simulink model "PID_MODEL"  (R2023b)
settings: Solver=FixedStepDiscrete  StartTime=0.0  StopTime=50  FixedStep=0.001  RelTol=1e-3
values from neighbouring files (symbols this model uses):
  ANG_A_D_CH1_1 = 0    [ini.m]
  ANG_A_D_CH1_2 = 0    [ini.m]
  ANG_A_D_CH1_3 = 0    [ini.m]
  ANG_A_D_CH1_4 = 0    [ini.m]
  ANG_A_D_CH1_5 = 0    [ini.m]
  ANG_A_D_CH1_6 = 0    [ini.m]
  ANG_A_D_CH1_7 = 0    [ini.m]
  ANG_A_D_CH2_1 = 0    [ini.m]
  ANG_A_D_CH2_2 = 0    [ini.m]
  ANG_A_D_CH2_3 = 0    [ini.m]
  ANG_A_D_CH2_4 = 0    [ini.m]
  ANG_A_D_CH2_5 = 0    [ini.m]
  ANG_A_D_CH2_6 = 0    [ini.m]
  ANG_A_D_CH2_7 = 0    [ini.m]
  ANG_A_I_CH1_1 = 0    [ini.m]
  ANG_A_I_CH1_2 = 0    [ini.m]
  ANG_A_I_CH1_3 = 0    [ini.m]
  ANG_A_I_CH1_4 = 0    [ini.m]
  ANG_A_I_CH1_5 = 0    [ini.m]
  ANG_A_I_CH1_6 = 0    [ini.m]
  ANG_A_I_CH1_7 = 0    [ini.m]
  ANG_A_I_CH2_1 = 0    [ini.m]
  ANG_A_I_CH2_2 = 0    [ini.m]
  ANG_A_I_CH2_3 = 0    [ini.m]
  ANG_A_I_CH2_4 = 0    [ini.m]
  ANG_A_I_CH2_5 = 0    [ini.m]
  ANG_A_I_CH2_6 = 0    [ini.m]
  ANG_A_I_CH2_7 = 0    [ini.m]
  ANG_A_P_CH1_1 = 0    [ini.m]
  ANG_A_P_CH1_2 = 0    [ini.m]
  ANG_A_P_CH1_3 = 0    [ini.m]
  ANG_A_P_CH1_4 = 0    [ini.m]
  ANG_A_P_CH1_5 = 0    [ini.m]
  ANG_A_P_CH1_6 = 0    [ini.m]
  ANG_A_P_CH1_7 = 0    [ini.m]
  ANG_A_P_CH2_1 = 0    [ini.m]
  ANG_A_P_CH2_2 = 0    [ini.m]
  ANG_A_P_CH2_3 = 0    [ini.m]
  ANG_A_P_CH2_4 = 0    [ini.m]
  ANG_A_P_CH2_5 = 0    [ini.m]
  ANG_A_P_CH2_6 = 0    [ini.m]
  ANG_A_P_CH2_7 = 0    [ini.m]
  ANG_S_D_CH1_1 = 0    [ini.m]
  ANG_S_D_CH1_2 = 0    [ini.m]
  ANG_S_D_CH1_3 = 0    [ini.m]
  ANG_S_D_CH1_4 = 0    [ini.m]
  ANG_S_D_CH1_5 = 0    [ini.m]
  ANG_S_D_CH1_6 = 0    [ini.m]
  ANG_S_D_CH1_7 = 0    [ini.m]
  ANG_S_D_CH2_1 = 0    [ini.m]
  ANG_S_D_CH2_2 = 0    [ini.m]
  ANG_S_D_CH2_3 = 0    [ini.m]
  ANG_S_D_CH2_4 = 0    [ini.m]
  ANG_S_D_CH2_5 = 0    [ini.m]
  ANG_S_D_CH2_6 = 0    [ini.m]
  ANG_S_D_CH2_7 = 0    [ini.m]
  ANG_S_I_CH1_1 = 0    [ini.m]
  ANG_S_I_CH1_2 = 0    [ini.m]
  ANG_S_I_CH1_3 = 0    [ini.m]
  ANG_S_I_CH1_4 = 0    [ini.m]
  ANG_S_I_CH1_5 = 0    [ini.m]
  ANG_S_I_CH1_6 = 0    [ini.m]
  ANG_S_I_CH1_7 = 0    [ini.m]
  ANG_S_I_CH2_1 = 0    [ini.m]
  ANG_S_I_CH2_2 = 0    [ini.m]
  ANG_S_I_CH2_3 = 0    [ini.m]
  ANG_S_I_CH2_4 = 0    [ini.m]
  ANG_S_I_CH2_5 = 0    [ini.m]
  ANG_S_I_CH2_6 = 0    [ini.m]
  ANG_S_I_CH2_7 = 0    [ini.m]
  ANG_S_P_CH1_1 = 0    [ini.m]
  ANG_S_P_CH1_2 = 0    [ini.m]
  ANG_S_P_CH1_3 = 0    [ini.m]
  ANG_S_P_CH1_4 = 0    [ini.m]
  ANG_S_P_CH1_5 = 0    [ini.m]
  ANG_S_P_CH1_6 = 0    [ini.m]
  ANG_S_P_CH1_7 = 0    [ini.m]
  ANG_S_P_CH2_1 = 0    [ini.m]
  ANG_S_P_CH2_2 = 0    [ini.m]
  ANG_S_P_CH2_3 = 0    [ini.m]
  ANG_S_P_CH2_4 = 0    [ini.m]
  ANG_S_P_CH2_5 = 0    [ini.m]
  ANG_S_P_CH2_6 = 0    [ini.m]
  ANG_S_P_CH2_7 = 0    [ini.m]
  DEADBAND_CH1_1 = 500    [ini.m]
  DEADBAND_CH1_2 = 500    [ini.m]
  DEADBAND_CH1_3 = 500    [ini.m]
  DEADBAND_CH1_4 = 500    [ini.m]
  DEADBAND_CH1_5 = 500    [ini.m]
  DEADBAND_CH1_6 = 500    [ini.m]
  DEADBAND_CH1_7 = 500    [ini.m]
  DEADBAND_CH2_1 = 500    [ini.m]
  DEADBAND_CH2_2 = 500    [ini.m]
  DEADBAND_CH2_3 = 500    [ini.m]
  DEADBAND_CH2_4 = 500    [ini.m]
  DEADBAND_CH2_5 = 500    [ini.m]
  DEADBAND_CH2_6 = 500    [ini.m]
  DEADBAND_CH2_7 = 500    [ini.m]
  SPD_D_CH1_1 = 0    [ini.m]
  SPD_D_CH1_2 = 0    [ini.m]
  SPD_D_CH1_3 = 0    [ini.m]
  SPD_D_CH1_4 = 0    [ini.m]
  SPD_D_CH1_5 = 0    [ini.m]
  SPD_D_CH1_6 = 0    [ini.m]
  SPD_D_CH1_7 = 0    [ini.m]
  SPD_D_CH2_1 = 0    [ini.m]
  SPD_D_CH2_2 = 0    [ini.m]
  SPD_D_CH2_3 = 0    [ini.m]
  SPD_D_CH2_4 = 0    [ini.m]
  SPD_D_CH2_5 = 0    [ini.m]
  SPD_D_CH2_6 = 0    [ini.m]
  SPD_D_CH2_7 = 0    [ini.m]
  SPD_I_CH1_1 = 0    [ini.m]
  SPD_I_CH1_2 = 0    [ini.m]
  SPD_I_CH1_3 = 0    [ini.m]
  SPD_I_CH1_4 = 0    [ini.m]
  SPD_I_CH1_5 = 0    [ini.m]
  SPD_I_CH1_6 = 0    [ini.m]
  SPD_I_CH1_7 = 0    [ini.m]
  SPD_I_CH2_1 = 0    [ini.m]
  ... (+34 more)
libraries: slpidlib x42
(part 1 of 5)
settings Model: TunableVars=ANG_A_D_CH1_1,ANG_A_D_CH1_2,ANG_A_D_CH1_3,ANG_A_D_CH1_4,ANG_A_D_CH1_5,ANG_A_D_CH1_6,ANG_A_D_CH1_7,ANG_A_D_CH2_1,ANG_A_D_CH2_2,ANG_A_D_CH2_3,ANG_A_D_CH2_4,ANG_A_D_CH2_5,ANG_A_D_CH2_6,ANG_A_D_CH2_7,ANG_A_I_CH1_1,ANG_A_I_CH1_2,ANG_A_I_CH1_3,ANG_A_I_CH1_4,ANG_A_I_CH1_5,ANG_A_I_CH1_6,ANG_A_I_CH1_7,ANG_A_I_CH2_1,ANG_A_I_CH2_2,ANG_A_I_CH2_3,ANG_A_I_CH2_4,ANG_A_I_CH2_5,ANG_A_I_CH2_6,ANG_A_I_CH2_7,ANG_A_P_CH1_1,ANG_A_P_CH1_2,ANG_A_P_CH1_3,ANG_A_P_CH1_4,ANG_A_P_CH1_5,ANG_A_P_CH1_6,ANG_A_P_CH1_7,ANG_A_P_CH2_1,ANG_A_P_CH2_2,ANG_A_P_CH2_3,ANG_A_P_CH2_4,ANG_A_P_CH2_5,ANG_A_P_CH2_6,ANG_A_P_CH2_7,ANG_S_D_CH1_1,ANG_S_D_CH1_2,ANG_S_D_CH1_3,ANG_S_D_CH1_4,ANG_S_D_CH1_5,ANG_S_D_CH1_6,ANG_S_D_CH1_7,ANG_S_D_CH2_1,ANG_S_D_CH2_2,ANG_S_D_CH2_3,ANG_S_D_CH2_4,ANG_S_D_CH2_5,ANG_S_D_CH2_6,ANG_S_D_CH2_7,ANG_S_I_CH1_1,ANG_S_I_CH1_2,ANG_S_I_CH1_3,ANG_S_I_CH1_4,ANG_S_I_CH1_5,ANG_S_I_CH1_6,ANG_S_I_CH1_7,ANG_S_I_CH2_1,ANG_S_I_CH2_2,ANG_S_I_CH2_3,ANG_S_I_CH2_4,ANG_S_I_CH2_5,ANG_S_I_CH2_6,ANG_S_I_CH2_7,ANG_S_P_CH1_1,ANG_S_P_CH1_2,ANG_S_P_CH1_3,ANG_S_P_CH1_4,ANG_S_P_CH1_5,ANG_S_P_CH1_6,ANG_S_P_CH1_7,ANG_S_P_CH2_1,ANG_S_P_CH2_2,ANG_S_P_CH2_3,ANG_S_P_CH2_4,ANG_S_P_CH2_5,ANG_S_P_CH2_6,ANG_S_P_CH2_7,DEADBAND_CH1_1,DEADBAND_CH1_2,DEADBAND_CH1_3,DEADBAND_CH1_4,DEADBAND_CH1_5,DEADBAND_CH1_6,DEADBAND_CH1_7,DEADBAND_CH2_1,DEADBAND_CH2_2,DEADBAND_CH2_3,DEADBAND_CH2_4,DEADBAND_CH2_5,DEADBAND_CH2_6,DEADBAND_CH2_7,SPD_D_CH1_1,SPD_D_CH1_2,SPD_D_CH1_3,SPD_D_CH1_4,SPD_D_CH1_5,SPD_D_CH1_6,SPD_D_CH1_7,SPD_D_CH2_1,SPD_D_CH2_2,SPD_D_CH2_3,SPD_D_CH2_4,SPD_D_CH2_5,SPD_D_CH2_6,SPD_D_CH2_7,SPD_I_CH1_1,SPD_I_CH1_2,SPD_I_CH1_3,SPD_I_CH1_4,SPD_I_CH1_5,SPD_I_CH1_6,SPD_I_CH1_7,SPD_I_CH2_1,SPD_I_CH2_2,SPD_I_CH2_3,SPD_I_CH2_4,SPD_I_CH2_5,SPD_I_CH2_6,SPD_I_CH2_7,SPD_P_CH1_1,SPD_P_CH1_2,SPD_P_CH1_3,SPD_P_CH1_4,SPD_P_CH1_5,SPD_P_CH1_6,SPD_P_CH1_7,SPD_P_CH2_1,SPD_P_CH2_2,SPD_P_CH2_3,SPD_P_CH2_4,SPD_P_CH2_5,SPD_P_CH2_6,SPD_P_CH2_7,TRANS_CH1_1,TRANS_CH1_2,TRANS_CH1_3,TRANS_CH1_4,TRANS_CH1_5,TRANS_CH1_6,TRANS_CH1_7,TRANS_CH2_1,TRANS_CH2_2,TRANS_CH2_3,TRANS_CH2_4,TRANS_CH2_5,TRANS_CH2_6,TRANS_CH2_7  TunableVarsStorageClass=Auto,Auto,Auto,Auto,Auto,Auto,Auto,Auto,Auto,Auto,Auto,Auto,Auto,Auto,Auto,Auto,Auto,Auto,Auto,Auto,Auto,Auto,Auto,Auto,Auto,Auto,Auto,Auto,Auto,Auto,Auto,Auto,Auto,Auto,Auto,Auto,Auto,Auto,Auto,Auto,Auto,Auto,Auto,Auto,Auto,Auto,Auto,Auto,Auto,Auto,Auto,Auto,Auto,Auto,Auto,Auto,Auto,Auto,Auto,Auto,Auto,Auto,Auto,Auto,Auto,Auto,Auto,Auto,Auto,Auto,Auto,Auto,Auto,Auto,Auto,Auto,Auto,Auto,Auto,Auto,Auto,Auto,Auto,Auto,Auto,Auto,Auto,Auto,Auto,Auto,Auto,Auto,Auto,Auto,Auto,Auto,Auto,Auto,Auto,Auto,Auto,Auto,Auto,Auto,Auto,Auto,Auto,Auto,Auto,Auto,Auto,Auto,Auto,Auto,Auto,Auto,Auto,Auto,Auto,Auto,Auto,Auto,Auto,Auto,Auto,Auto,Auto,Auto,Auto,Auto,Auto,Auto,Auto,Auto,Auto,Auto,Auto,Auto,Auto,Auto,Auto,Auto,Auto,Auto,Auto,Auto,Auto,Auto,Auto,Auto,Auto,Auto,Auto,Auto  TunableVarsTypeQualifier=,,,,,,,,,,,,,,,,,,,,,,,,,,,,,,,,,,,,,,,,,,,,,,,,,,,,,,,,,,,,,,,,,,,,,,,,,,,,,,,,,,,,,,,,,,,,,,,,,,,,,,,,,,,,,,,,,,,,,,,,,,,,,,,,,,,,,,,,,,,,,,,,,,,,,,,,,  Creator=james  LastModifiedBy=12697
settings OptimizationCC: DefaultParameterBehavior=Inlined  UseDivisionForNetSlopeComputation=on  GainParamInheritBuiltInType=on  UseFloatMulNetSlope=on  InlineInvariantSignals=on  PassReuseOutputArgsAs=Individual arguments  ZeroExternalMemoryAtStartup=off  ZeroInternalMemoryAtStartup=off  NoFixptDivByZeroProtection=on  EfficientFloat2IntCast=on  LifeSpan=1  MaxStackSize=64  OptimizeBlockOrder=speed  DifferentSizesBufferReuse=on  EfficientTunableParamExpr=on
settings DebuggingCC: ParameterTunabilityLossMsg=error
settings HardwareCC: ProdBitPerPointer=32  ProdBitPerSizeT=32  ProdBitPerPtrDiffT=32  ProdLargestAtomicInteger=Long  ProdLargestAtomicFloat=Double  ProdWordSize=32  ProdLongLongMode=on  ProdHWDeviceType=ARM Compatible->ARM Cortex-M
settings SFSimCC: MATLABDynamicMemAlloc=off
settings RTWCC: Description=Embedded Coder  SystemTargetFile=ert.tlc  GenCodeOnly=on  TemplateMakefile=ert_default_tmf  GenerateReport=on  Toolchain=GNU Tools for ARM Embedded Processors  LaunchReport=on
settings CodeAppCC: ForceParamTrailComments=on  IgnoreCustomStorageClasses=off  OperatorAnnotations=on  SimulinkDataObjDesc=on  SFDataObjDesc=on  CustomSymbolStrGlobalVar=rt$N$M  CustomSymbolStrType=$N$M  CustomSymbolStrFcn=$N$M$F  CustomSymbolStrMacro=$N$M  InsertBlockDesc=on
settings ERTTargetCC: CodeReplacementLibrary=ARM Cortex-M  IncludeMdlTerminateFcn=off  CombineSignalStateStructs=on  SupportAbsoluteTime=off  SupportComplex=off  SupportNonInlinedSFcns=on  InlinedParameterPlacement=NonHierarchical  ERTCustomFileTemplate=example_file_process.tlc  ERTFilePackagingFormat=CompactWithDataFile

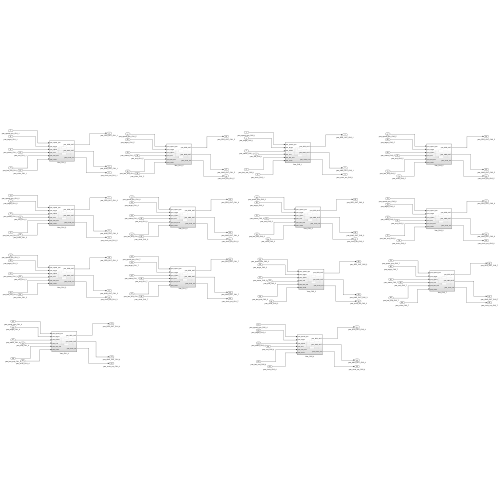
[thumbnail: Simulink's stored preview of the top-level diagram]
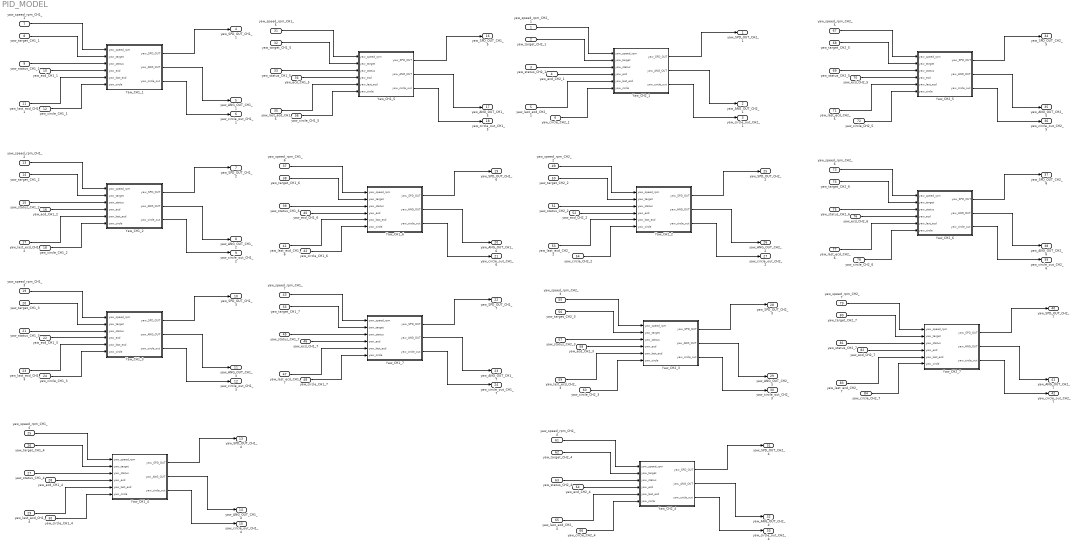
== system PID_MODEL ==
  yaw_speed_rpm_CH2_1 : Inport  OutDataTypeStr=single
  yaw_target_CH2_1 : Inport  Port=2  OutDataTypeStr=single
  yaw_status_CH2_1 : Inport  Port=3  OutDataTypeStr=single
  yaw_ecd_CH2_1 : Inport  Port=4  OutDataTypeStr=single
  yaw_last_ecd_CH2_1 : Inport  Port=5  OutDataTypeStr=single
  yaw_circle_CH2_1 : Inport  Port=6  OutDataTypeStr=single
  yaw_speed_rpm_CH1_1 : Inport  Port=7  OutDataTypeStr=single
  yaw_target_CH1_1 : Inport  Port=8  OutDataTypeStr=single
  yaw_status_CH1_1 : Inport  Port=9  OutDataTypeStr=single
  yaw_ecd_CH1_1 : Inport  Port=10  OutDataTypeStr=single
  yaw_last_ecd_CH1_1 : Inport  Port=11  OutDataTypeStr=single
  yaw_circle_CH1_1 : Inport  Port=12  OutDataTypeStr=single
  yaw_speed_rpm_CH1_2 : Inport  Port=13  OutDataTypeStr=single
  yaw_target_CH1_2 : Inport  Port=14  OutDataTypeStr=single
  yaw_status_CH1_2 : Inport  Port=15  OutDataTypeStr=single
  yaw_ecd_CH1_2 : Inport  Port=16  OutDataTypeStr=single
  yaw_last_ecd_CH1_2 : Inport  Port=17  OutDataTypeStr=single
  yaw_circle_CH1_2 : Inport  Port=18  OutDataTypeStr=single
  yaw_speed_rpm_CH1_3 : Inport  Port=19  OutDataTypeStr=single
  yaw_target_CH1_3 : Inport  Port=20  OutDataTypeStr=single
  yaw_status_CH1_3 : Inport  Port=21  OutDataTypeStr=single
  yaw_ecd_CH1_3 : Inport  Port=22  OutDataTypeStr=single
  yaw_last_ecd_CH1_3 : Inport  Port=23  OutDataTypeStr=single
  yaw_circle_CH1_3 : Inport  Port=24  OutDataTypeStr=single
  yaw_speed_rpm_CH1_4 : Inport  Port=25  OutDataTypeStr=single
  yaw_target_CH1_4 : Inport  Port=26  OutDataTypeStr=single
  yaw_status_CH1_4 : Inport  Port=27  OutDataTypeStr=single
  yaw_ecd_CH1_4 : Inport  Port=28  OutDataTypeStr=single
  yaw_last_ecd_CH1_4 : Inport  Port=29  OutDataTypeStr=single
  yaw_circle_CH1_4 : Inport  Port=30  OutDataTypeStr=single
  yaw_speed_rpm_CH1_5 : Inport  Port=31  OutDataTypeStr=single
  yaw_target_CH1_5 : Inport  Port=32  OutDataTypeStr=single
  yaw_status_CH1_5 : Inport  Port=33  OutDataTypeStr=single
  yaw_ecd_CH1_5 : Inport  Port=34  OutDataTypeStr=single
  yaw_last_ecd_CH1_5 : Inport  Port=35  OutDataTypeStr=single
  yaw_circle_CH1_5 : Inport  Port=36  OutDataTypeStr=single
  yaw_speed_rpm_CH1_6 : Inport  Port=37  OutDataTypeStr=single
  yaw_target_CH1_6 : Inport  Port=38  OutDataTypeStr=single
  yaw_status_CH1_6 : Inport  Port=39  OutDataTypeStr=single
  yaw_ecd_CH1_6 : Inport  Port=40  OutDataTypeStr=single
  yaw_last_ecd_CH1_6 : Inport  Port=41  OutDataTypeStr=single
  yaw_circle_CH1_6 : Inport  Port=42  OutDataTypeStr=single
  yaw_speed_rpm_CH1_7 : Inport  Port=43  OutDataTypeStr=single
  yaw_target_CH1_7 : Inport  Port=44  OutDataTypeStr=single
  yaw_status_CH1_7 : Inport  Port=45  OutDataTypeStr=single
  yaw_ecd_CH1_7 : Inport  Port=46  OutDataTypeStr=single
  yaw_last_ecd_CH1_7 : Inport  Port=47  OutDataTypeStr=single
  yaw_circle_CH1_7 : Inport  Port=48  OutDataTypeStr=single
  yaw_speed_rpm_CH2_2 : Inport  Port=49  OutDataTypeStr=single
  yaw_target_CH2_2 : Inport  Port=50  OutDataTypeStr=single
  yaw_status_CH2_2 : Inport  Port=51  OutDataTypeStr=single
  yaw_ecd_CH2_2 : Inport  Port=52  OutDataTypeStr=single
  yaw_last_ecd_CH2_2 : Inport  Port=53  OutDataTypeStr=single
  yaw_circle_CH2_2 : Inport  Port=54  OutDataTypeStr=single
  yaw_speed_rpm_CH2_3 : Inport  Port=55  OutDataTypeStr=single
  yaw_target_CH2_3 : Inport  Port=56  OutDataTypeStr=single
  yaw_status_CH2_3 : Inport  Port=57  OutDataTypeStr=single
  yaw_ecd_CH2_3 : Inport  Port=58  OutDataTypeStr=single
  yaw_last_ecd_CH2_3 : Inport  Port=59  OutDataTypeStr=single
  yaw_circle_CH2_3 : Inport  Port=60  OutDataTypeStr=single
  yaw_speed_rpm_CH2_4 : Inport  Port=61  OutDataTypeStr=single
  yaw_target_CH2_4 : Inport  Port=62  OutDataTypeStr=single
  yaw_status_CH2_4 : Inport  Port=63  OutDataTypeStr=single
  yaw_ecd_CH2_4 : Inport  Port=64  OutDataTypeStr=single
  yaw_last_ecd_CH2_4 : Inport  Port=65  OutDataTypeStr=single
  yaw_circle_CH2_4 : Inport  Port=66  OutDataTypeStr=single
  yaw_speed_rpm_CH2_5 : Inport  Port=67  OutDataTypeStr=single
  yaw_target_CH2_5 : Inport  Port=68  OutDataTypeStr=single
  yaw_status_CH2_5 : Inport  Port=69  OutDataTypeStr=single
  yaw_ecd_CH2_5 : Inport  Port=70  OutDataTypeStr=single
  yaw_last_ecd_CH2_5 : Inport  Port=71  OutDataTypeStr=single
  yaw_circle_CH2_5 : Inport  Port=72  OutDataTypeStr=single
  yaw_speed_rpm_CH2_6 : Inport  Port=73  OutDataTypeStr=single
  yaw_target_CH2_6 : Inport  Port=74  OutDataTypeStr=single
  yaw_status_CH2_6 : Inport  Port=75  OutDataTypeStr=single
  yaw_ecd_CH2_6 : Inport  Port=76  OutDataTypeStr=single
  yaw_last_ecd_CH2_6 : Inport  Port=77  OutDataTypeStr=single
  yaw_circle_CH2_6 : Inport  Port=78  OutDataTypeStr=single
  yaw_speed_rpm_CH2_7 : Inport  Port=79  OutDataTypeStr=single
  yaw_target_CH2_7 : Inport  Port=80  OutDataTypeStr=single
  yaw_status_CH2_7 : Inport  Port=81  OutDataTypeStr=single
  yaw_ecd_CH2_7 : Inport  Port=82  OutDataTypeStr=single
  yaw_last_ecd_CH2_7 : Inport  Port=83  OutDataTypeStr=single
  yaw_circle_CH2_7 : Inport  Port=84  OutDataTypeStr=single
  Yaw_CH1_1 : Subsystem
  Yaw_CH1_2 : Subsystem
  Yaw_CH1_3 : Subsystem
  Yaw_CH1_4 : Subsystem
  Yaw_CH1_5 : Subsystem
  Yaw_CH1_6 : Subsystem
  Yaw_CH1_7 : Subsystem
  Yaw_CH2_1 : Subsystem
  Yaw_CH2_2 : Subsystem
  Yaw_CH2_3 : Subsystem
  Yaw_CH2_4 : Subsystem
  Yaw_CH2_5 : Subsystem
  Yaw_CH2_6 : Subsystem
  Yaw_CH2_7 : Subsystem
  yaw_SPD_OUT_CH2_1 : Outport  OutDataTypeStr=single
  yaw_ANG_OUT_CH2_1 : Outport  Port=2  OutDataTypeStr=single
  yaw_circle_out_CH2_1 : Outport  Port=3  OutDataTypeStr=single
  yaw_SPD_OUT_CH1_1 : Outport  Port=4  OutDataTypeStr=single
  yaw_ANG_OUT_CH1_1 : Outport  Port=5  OutDataTypeStr=single
  yaw_circle_out_CH1_1 : Outport  Port=6  OutDataTypeStr=single
  yaw_SPD_OUT_CH1_2 : Outport  Port=7  OutDataTypeStr=single
  yaw_ANG_OUT_CH1_2 : Outport  Port=8  OutDataTypeStr=single
  yaw_circle_out_CH1_2 : Outport  Port=9  OutDataTypeStr=single
  yaw_SPD_OUT_CH1_3 : Outport  Port=10  OutDataTypeStr=single
  yaw_ANG_OUT_CH1_3 : Outport  Port=11  OutDataTypeStr=single
  yaw_circle_out_CH1_3 : Outport  Port=12  OutDataTypeStr=single
  yaw_SPD_OUT_CH1_4 : Outport  Port=13  OutDataTypeStr=single
  yaw_ANG_OUT_CH1_4 : Outport  Port=14  OutDataTypeStr=single
  yaw_circle_out_CH1_4 : Outport  Port=15  OutDataTypeStr=single
  yaw_SPD_OUT_CH1_5 : Outport  Port=16  OutDataTypeStr=single
  yaw_ANG_OUT_CH1_5 : Outport  Port=17  OutDataTypeStr=single
  yaw_circle_out_CH1_5 : Outport  Port=18  OutDataTypeStr=single
  yaw_SPD_OUT_CH1_6 : Outport  Port=19  OutDataTypeStr=single
  yaw_ANG_OUT_CH1_6 : Outport  Port=20  OutDataTypeStr=single
  yaw_circle_out_CH1_6 : Outport  Port=21  OutDataTypeStr=single
  yaw_SPD_OUT_CH1_7 : Outport  Port=22  OutDataTypeStr=single
  yaw_ANG_OUT_CH1_7 : Outport  Port=23  OutDataTypeStr=single
  yaw_circle_out_CH1_7 : Outport  Port=24  OutDataTypeStr=single
  yaw_SPD_OUT_CH2_2 : Outport  Port=25  OutDataTypeStr=single
  yaw_ANG_OUT_CH2_2 : Outport  Port=26  OutDataTypeStr=single
  yaw_circle_out_CH2_2 : Outport  Port=27  OutDataTypeStr=single
  yaw_SPD_OUT_CH2_3 : Outport  Port=28  OutDataTypeStr=single
  yaw_ANG_OUT_CH2_3 : Outport  Port=29  OutDataTypeStr=single
  yaw_circle_out_CH2_3 : Outport  Port=30  OutDataTypeStr=single
  yaw_SPD_OUT_CH2_4 : Outport  Port=31  OutDataTypeStr=single
  yaw_ANG_OUT_CH2_4 : Outport  Port=32  OutDataTypeStr=single
  yaw_circle_out_CH2_4 : Outport  Port=33  OutDataTypeStr=single
  yaw_SPD_OUT_CH2_5 : Outport  Port=34  OutDataTypeStr=single
  yaw_ANG_OUT_CH2_5 : Outport  Port=35  OutDataTypeStr=single
  yaw_circle_out_CH2_5 : Outport  Port=36  OutDataTypeStr=single
  yaw_SPD_OUT_CH2_6 : Outport  Port=37  OutDataTypeStr=single
  yaw_ANG_OUT_CH2_6 : Outport  Port=38  OutDataTypeStr=single
  yaw_circle_out_CH2_6 : Outport  Port=39  OutDataTypeStr=single
  yaw_SPD_OUT_CH2_7 : Outport  Port=40  OutDataTypeStr=single
  yaw_ANG_OUT_CH2_7 : Outport  Port=41  OutDataTypeStr=single
  yaw_circle_out_CH2_7 : Outport  Port=42  OutDataTypeStr=single
  wires:
  Yaw_CH2_1/2(yaw_ANG_OUT) -> yaw_ANG_OUT_CH2_1/1
  yaw_speed_rpm_CH2_1/1 -> Yaw_CH2_1/1(yaw_speed_rpm)
  yaw_last_ecd_CH2_1/1 -> Yaw_CH2_1/5(yaw_last_ecd)
  yaw_circle_CH2_1/1 -> Yaw_CH2_1/6(yaw_circle)
  yaw_target_CH2_1/1 -> Yaw_CH2_1/2(yaw_target)
  Yaw_CH2_1/1(yaw_SPD_OUT) -> yaw_SPD_OUT_CH2_1/1
  yaw_ecd_CH2_1/1 -> Yaw_CH2_1/4(yaw_ecd)
  yaw_status_CH2_1/1 -> Yaw_CH2_1/3(yaw_status)
  Yaw_CH2_1/3(yaw_circle_out) -> yaw_circle_out_CH2_1/1
  Yaw_CH1_1/3(yaw_circle_out) -> yaw_circle_out_CH1_1/1
  yaw_speed_rpm_CH1_1/1 -> Yaw_CH1_1/1(yaw_speed_rpm)
  Yaw_CH1_1/1(yaw_SPD_OUT) -> yaw_SPD_OUT_CH1_1/1
  yaw_circle_CH1_1/1 -> Yaw_CH1_1/6(yaw_circle)
  yaw_ecd_CH1_1/1 -> Yaw_CH1_1/4(yaw_ecd)
  yaw_target_CH1_1/1 -> Yaw_CH1_1/2(yaw_target)
  yaw_last_ecd_CH1_1/1 -> Yaw_CH1_1/5(yaw_last_ecd)
  yaw_status_CH1_1/1 -> Yaw_CH1_1/3(yaw_status)
  Yaw_CH1_1/2(yaw_ANG_OUT) -> yaw_ANG_OUT_CH1_1/1
  yaw_status_CH1_2/1 -> Yaw_CH1_2/3(yaw_status)
  Yaw_CH1_2/2(yaw_ANG_OUT) -> yaw_ANG_OUT_CH1_2/1
  yaw_circle_CH1_2/1 -> Yaw_CH1_2/6(yaw_circle)
  yaw_ecd_CH1_2/1 -> Yaw_CH1_2/4(yaw_ecd)
  Yaw_CH1_2/3(yaw_circle_out) -> yaw_circle_out_CH1_2/1
  yaw_speed_rpm_CH1_2/1 -> Yaw_CH1_2/1(yaw_speed_rpm)
  yaw_last_ecd_CH1_2/1 -> Yaw_CH1_2/5(yaw_last_ecd)
  Yaw_CH1_2/1(yaw_SPD_OUT) -> yaw_SPD_OUT_CH1_2/1
  yaw_target_CH1_2/1 -> Yaw_CH1_2/2(yaw_target)
  yaw_status_CH1_3/1 -> Yaw_CH1_3/3(yaw_status)
  Yaw_CH1_3/2(yaw_ANG_OUT) -> yaw_ANG_OUT_CH1_3/1
  yaw_circle_CH1_3/1 -> Yaw_CH1_3/6(yaw_circle)
  yaw_ecd_CH1_3/1 -> Yaw_CH1_3/4(yaw_ecd)
  Yaw_CH1_3/3(yaw_circle_out) -> yaw_circle_out_CH1_3/1
  yaw_speed_rpm_CH1_3/1 -> Yaw_CH1_3/1(yaw_speed_rpm)
  yaw_last_ecd_CH1_3/1 -> Yaw_CH1_3/5(yaw_last_ecd)
  Yaw_CH1_3/1(yaw_SPD_OUT) -> yaw_SPD_OUT_CH1_3/1
  yaw_target_CH1_3/1 -> Yaw_CH1_3/2(yaw_target)
  yaw_status_CH1_4/1 -> Yaw_CH1_4/3(yaw_status)
  Yaw_CH1_4/2(yaw_ANG_OUT) -> yaw_ANG_OUT_CH1_4/1
  yaw_circle_CH1_4/1 -> Yaw_CH1_4/6(yaw_circle)
  yaw_ecd_CH1_4/1 -> Yaw_CH1_4/4(yaw_ecd)
  Yaw_CH1_4/3(yaw_circle_out) -> yaw_circle_out_CH1_4/1
  yaw_speed_rpm_CH1_4/1 -> Yaw_CH1_4/1(yaw_speed_rpm)
  yaw_last_ecd_CH1_4/1 -> Yaw_CH1_4/5(yaw_last_ecd)
  Yaw_CH1_4/1(yaw_SPD_OUT) -> yaw_SPD_OUT_CH1_4/1
  yaw_target_CH1_4/1 -> Yaw_CH1_4/2(yaw_target)
  yaw_status_CH1_5/1 -> Yaw_CH1_5/3(yaw_status)
  Yaw_CH1_5/2(yaw_ANG_OUT) -> yaw_ANG_OUT_CH1_5/1
  yaw_circle_CH1_5/1 -> Yaw_CH1_5/6(yaw_circle)
  yaw_ecd_CH1_5/1 -> Yaw_CH1_5/4(yaw_ecd)
  Yaw_CH1_5/3(yaw_circle_out) -> yaw_circle_out_CH1_5/1
  yaw_speed_rpm_CH1_5/1 -> Yaw_CH1_5/1(yaw_speed_rpm)
  yaw_last_ecd_CH1_5/1 -> Yaw_CH1_5/5(yaw_last_ecd)
  Yaw_CH1_5/1(yaw_SPD_OUT) -> yaw_SPD_OUT_CH1_5/1
  yaw_target_CH1_5/1 -> Yaw_CH1_5/2(yaw_target)
  yaw_status_CH1_6/1 -> Yaw_CH1_6/3(yaw_status)
  Yaw_CH1_6/2(yaw_ANG_OUT) -> yaw_ANG_OUT_CH1_6/1
  yaw_circle_CH1_6/1 -> Yaw_CH1_6/6(yaw_circle)
  yaw_ecd_CH1_6/1 -> Yaw_CH1_6/4(yaw_ecd)
  Yaw_CH1_6/3(yaw_circle_out) -> yaw_circle_out_CH1_6/1
  yaw_speed_rpm_CH1_6/1 -> Yaw_CH1_6/1(yaw_speed_rpm)
  yaw_last_ecd_CH1_6/1 -> Yaw_CH1_6/5(yaw_last_ecd)
  Yaw_CH1_6/1(yaw_SPD_OUT) -> yaw_SPD_OUT_CH1_6/1
  yaw_target_CH1_6/1 -> Yaw_CH1_6/2(yaw_target)
  yaw_status_CH1_7/1 -> Yaw_CH1_7/3(yaw_status)
  Yaw_CH1_7/2(yaw_ANG_OUT) -> yaw_ANG_OUT_CH1_7/1
  yaw_circle_CH1_7/1 -> Yaw_CH1_7/6(yaw_circle)
  yaw_ecd_CH1_7/1 -> Yaw_CH1_7/4(yaw_ecd)
  Yaw_CH1_7/3(yaw_circle_out) -> yaw_circle_out_CH1_7/1
  yaw_speed_rpm_CH1_7/1 -> Yaw_CH1_7/1(yaw_speed_rpm)
  yaw_last_ecd_CH1_7/1 -> Yaw_CH1_7/5(yaw_last_ecd)
  Yaw_CH1_7/1(yaw_SPD_OUT) -> yaw_SPD_OUT_CH1_7/1
  yaw_target_CH1_7/1 -> Yaw_CH1_7/2(yaw_target)
  yaw_circle_CH2_2/1 -> Yaw_CH2_2/6(yaw_circle)
  Yaw_CH2_2/1(yaw_SPD_OUT) -> yaw_SPD_OUT_CH2_2/1
  yaw_status_CH2_2/1 -> Yaw_CH2_2/3(yaw_status)
  yaw_target_CH2_2/1 -> Yaw_CH2_2/2(yaw_target)
  yaw_speed_rpm_CH2_2/1 -> Yaw_CH2_2/1(yaw_speed_rpm)
  yaw_ecd_CH2_2/1 -> Yaw_CH2_2/4(yaw_ecd)
  Yaw_CH2_2/3(yaw_circle_out) -> yaw_circle_out_CH2_2/1
  Yaw_CH2_2/2(yaw_ANG_OUT) -> yaw_ANG_OUT_CH2_2/1
  yaw_last_ecd_CH2_2/1 -> Yaw_CH2_2/5(yaw_last_ecd)
  yaw_circle_CH2_3/1 -> Yaw_CH2_3/6(yaw_circle)
  Yaw_CH2_3/1(yaw_SPD_OUT) -> yaw_SPD_OUT_CH2_3/1
  yaw_status_CH2_3/1 -> Yaw_CH2_3/3(yaw_status)
  yaw_target_CH2_3/1 -> Yaw_CH2_3/2(yaw_target)
  yaw_speed_rpm_CH2_3/1 -> Yaw_CH2_3/1(yaw_speed_rpm)
  yaw_ecd_CH2_3/1 -> Yaw_CH2_3/4(yaw_ecd)
  Yaw_CH2_3/3(yaw_circle_out) -> yaw_circle_out_CH2_3/1
  Yaw_CH2_3/2(yaw_ANG_OUT) -> yaw_ANG_OUT_CH2_3/1
  yaw_last_ecd_CH2_3/1 -> Yaw_CH2_3/5(yaw_last_ecd)
  yaw_circle_CH2_4/1 -> Yaw_CH2_4/6(yaw_circle)
  Yaw_CH2_4/1(yaw_SPD_OUT) -> yaw_SPD_OUT_CH2_4/1
  yaw_status_CH2_4/1 -> Yaw_CH2_4/3(yaw_status)
  yaw_target_CH2_4/1 -> Yaw_CH2_4/2(yaw_target)
  yaw_speed_rpm_CH2_4/1 -> Yaw_CH2_4/1(yaw_speed_rpm)
  yaw_ecd_CH2_4/1 -> Yaw_CH2_4/4(yaw_ecd)
  Yaw_CH2_4/3(yaw_circle_out) -> yaw_circle_out_CH2_4/1
  Yaw_CH2_4/2(yaw_ANG_OUT) -> yaw_ANG_OUT_CH2_4/1
  yaw_last_ecd_CH2_4/1 -> Yaw_CH2_4/5(yaw_last_ecd)
  yaw_circle_CH2_5/1 -> Yaw_CH2_5/6(yaw_circle)
  Yaw_CH2_5/1(yaw_SPD_OUT) -> yaw_SPD_OUT_CH2_5/1
  yaw_status_CH2_5/1 -> Yaw_CH2_5/3(yaw_status)
  yaw_target_CH2_5/1 -> Yaw_CH2_5/2(yaw_target)
  yaw_speed_rpm_CH2_5/1 -> Yaw_CH2_5/1(yaw_speed_rpm)
  yaw_ecd_CH2_5/1 -> Yaw_CH2_5/4(yaw_ecd)
  Yaw_CH2_5/3(yaw_circle_out) -> yaw_circle_out_CH2_5/1
  Yaw_CH2_5/2(yaw_ANG_OUT) -> yaw_ANG_OUT_CH2_5/1
  yaw_last_ecd_CH2_5/1 -> Yaw_CH2_5/5(yaw_last_ecd)
  yaw_circle_CH2_6/1 -> Yaw_CH2_6/6(yaw_circle)
  Yaw_CH2_6/1(yaw_SPD_OUT) -> yaw_SPD_OUT_CH2_6/1
  yaw_status_CH2_6/1 -> Yaw_CH2_6/3(yaw_status)
  yaw_target_CH2_6/1 -> Yaw_CH2_6/2(yaw_target)
  yaw_speed_rpm_CH2_6/1 -> Yaw_CH2_6/1(yaw_speed_rpm)
  yaw_ecd_CH2_6/1 -> Yaw_CH2_6/4(yaw_ecd)
  Yaw_CH2_6/3(yaw_circle_out) -> yaw_circle_out_CH2_6/1
  Yaw_CH2_6/2(yaw_ANG_OUT) -> yaw_ANG_OUT_CH2_6/1
  yaw_last_ecd_CH2_6/1 -> Yaw_CH2_6/5(yaw_last_ecd)
  yaw_circle_CH2_7/1 -> Yaw_CH2_7/6(yaw_circle)
  Yaw_CH2_7/1(yaw_SPD_OUT) -> yaw_SPD_OUT_CH2_7/1
  yaw_status_CH2_7/1 -> Yaw_CH2_7/3(yaw_status)
  yaw_target_CH2_7/1 -> Yaw_CH2_7/2(yaw_target)
  yaw_speed_rpm_CH2_7/1 -> Yaw_CH2_7/1(yaw_speed_rpm)
  yaw_ecd_CH2_7/1 -> Yaw_CH2_7/4(yaw_ecd)
  Yaw_CH2_7/3(yaw_circle_out) -> yaw_circle_out_CH2_7/1
  Yaw_CH2_7/2(yaw_ANG_OUT) -> yaw_ANG_OUT_CH2_7/1
  yaw_last_ecd_CH2_7/1 -> Yaw_CH2_7/5(yaw_last_ecd)

== system PID_MODEL/Yaw_CH1_1 ==
  yaw_speed_rpm : Inport  OutDataTypeStr=single
  yaw_target : Inport  Port=2  OutDataTypeStr=single
  yaw_status : Inport  Port=3  OutDataTypeStr=single
  yaw_ecd : Inport  Port=4  OutDataTypeStr=single
  yaw_last_ecd : Inport  Port=5  OutDataTypeStr=single
  yaw_circle : Inport  Port=6  OutDataTypeStr=single
  If Action_speed Subsystem : Subsystem  TreatAsAtomicUnit=on
  If Action_speed Subsystem1 : Subsystem  TreatAsAtomicUnit=on
  Switch Case : SwitchCase  CaseConditions={1,2}  ShowDefaultCase=off
  yaw_SPD_OUT : Outport  OutDataTypeStr=single
  yaw_ANG_OUT : Outport  Port=2  OutDataTypeStr=single
  yaw_circle_out : Outport  Port=3  OutDataTypeStr=single
  wires:
  Switch Case/1 -> If Action_speed Subsystem/Action
  yaw_speed_rpm/1 -> If Action_speed Subsystem1/1(yaw_speed_rpm), If Action_speed Subsystem/1(yaw_speed_rpm)
  yaw_target/1 -> If Action_speed Subsystem1/2(yaw_target), If Action_speed Subsystem/2(yaw_target)
  Switch Case/2 -> If Action_speed Subsystem1/Action
  yaw_ecd/1 -> If Action_speed Subsystem1/3(yaw_ecd)
  yaw_last_ecd/1 -> If Action_speed Subsystem1/4(yaw_last_ecd)
  If Action_speed Subsystem1/2(yaw_circle_out) -> yaw_circle_out/1
  yaw_status/1 -> Switch Case/1
  yaw_circle/1 -> If Action_speed Subsystem1/5(yaw_circle)
  If Action_speed Subsystem/1(Out1) -> yaw_SPD_OUT/1
  If Action_speed Subsystem1/1(Out1) -> yaw_ANG_OUT/1

== system PID_MODEL/Yaw_CH1_2 ==
  yaw_speed_rpm : Inport  OutDataTypeStr=single
  yaw_target : Inport  Port=2  OutDataTypeStr=single
  yaw_status : Inport  Port=3  OutDataTypeStr=single
  yaw_ecd : Inport  Port=4  OutDataTypeStr=single
  yaw_last_ecd : Inport  Port=5  OutDataTypeStr=single
  yaw_circle : Inport  Port=6  OutDataTypeStr=single
  If Action_speed Subsystem : Subsystem  TreatAsAtomicUnit=on
  If Action_speed Subsystem1 : Subsystem  TreatAsAtomicUnit=on
  Switch Case : SwitchCase  CaseConditions={1,2}  ShowDefaultCase=off
  yaw_SPD_OUT : Outport  OutDataTypeStr=single
  yaw_ANG_OUT : Outport  Port=2  OutDataTypeStr=single
  yaw_circle_out : Outport  Port=3  OutDataTypeStr=single
  wires:
  Switch Case/1 -> If Action_speed Subsystem/Action
  yaw_speed_rpm/1 -> If Action_speed Subsystem1/1(yaw_speed_rpm), If Action_speed Subsystem/1(yaw_speed_rpm)
  yaw_target/1 -> If Action_speed Subsystem1/2(yaw_target), If Action_speed Subsystem/2(yaw_target)
  Switch Case/2 -> If Action_speed Subsystem1/Action
  yaw_ecd/1 -> If Action_speed Subsystem1/3(yaw_ecd)
  yaw_last_ecd/1 -> If Action_speed Subsystem1/4(yaw_last_ecd)
  If Action_speed Subsystem1/2(yaw_circle_out) -> yaw_circle_out/1
  yaw_status/1 -> Switch Case/1
  yaw_circle/1 -> If Action_speed Subsystem1/5(yaw_circle)
  If Action_speed Subsystem/1(Out1) -> yaw_SPD_OUT/1
  If Action_speed Subsystem1/1(Out1) -> yaw_ANG_OUT/1

== system PID_MODEL/Yaw_CH1_3 ==
  yaw_speed_rpm : Inport  OutDataTypeStr=single
  yaw_target : Inport  Port=2  OutDataTypeStr=single
  yaw_status : Inport  Port=3  OutDataTypeStr=single
  yaw_ecd : Inport  Port=4  OutDataTypeStr=single
  yaw_last_ecd : Inport  Port=5  OutDataTypeStr=single
  yaw_circle : Inport  Port=6  OutDataTypeStr=single
  If Action_speed Subsystem : Subsystem  TreatAsAtomicUnit=on
  If Action_speed Subsystem1 : Subsystem  TreatAsAtomicUnit=on
  Switch Case : SwitchCase  CaseConditions={1,2}  ShowDefaultCase=off
  yaw_SPD_OUT : Outport  OutDataTypeStr=single
  yaw_ANG_OUT : Outport  Port=2  OutDataTypeStr=single
  yaw_circle_out : Outport  Port=3  OutDataTypeStr=single
  wires:
  Switch Case/1 -> If Action_speed Subsystem/Action
  yaw_speed_rpm/1 -> If Action_speed Subsystem1/1(yaw_speed_rpm), If Action_speed Subsystem/1(yaw_speed_rpm)
  yaw_target/1 -> If Action_speed Subsystem1/2(yaw_target), If Action_speed Subsystem/2(yaw_target)
  Switch Case/2 -> If Action_speed Subsystem1/Action
  yaw_ecd/1 -> If Action_speed Subsystem1/3(yaw_ecd)
  yaw_last_ecd/1 -> If Action_speed Subsystem1/4(yaw_last_ecd)
  If Action_speed Subsystem1/2(yaw_circle_out) -> yaw_circle_out/1
  yaw_status/1 -> Switch Case/1
  yaw_circle/1 -> If Action_speed Subsystem1/5(yaw_circle)
  If Action_speed Subsystem/1(Out1) -> yaw_SPD_OUT/1
  If Action_speed Subsystem1/1(Out1) -> yaw_ANG_OUT/1

== system PID_MODEL/Yaw_CH1_4 ==
  yaw_speed_rpm : Inport  OutDataTypeStr=single
  yaw_target : Inport  Port=2  OutDataTypeStr=single
  yaw_status : Inport  Port=3  OutDataTypeStr=single
  yaw_ecd : Inport  Port=4  OutDataTypeStr=single
  yaw_last_ecd : Inport  Port=5  OutDataTypeStr=single
  yaw_circle : Inport  Port=6  OutDataTypeStr=single
  If Action_speed Subsystem : Subsystem  TreatAsAtomicUnit=on
  If Action_speed Subsystem1 : Subsystem  TreatAsAtomicUnit=on
  Switch Case : SwitchCase  CaseConditions={1,2}  ShowDefaultCase=off
  yaw_SPD_OUT : Outport  OutDataTypeStr=single
  yaw_ANG_OUT : Outport  Port=2  OutDataTypeStr=single
  yaw_circle_out : Outport  Port=3  OutDataTypeStr=single
  wires:
  Switch Case/1 -> If Action_speed Subsystem/Action
  yaw_speed_rpm/1 -> If Action_speed Subsystem1/1(yaw_speed_rpm), If Action_speed Subsystem/1(yaw_speed_rpm)
  yaw_target/1 -> If Action_speed Subsystem1/2(yaw_target), If Action_speed Subsystem/2(yaw_target)
  Switch Case/2 -> If Action_speed Subsystem1/Action
  yaw_ecd/1 -> If Action_speed Subsystem1/3(yaw_ecd)
  yaw_last_ecd/1 -> If Action_speed Subsystem1/4(yaw_last_ecd)
  If Action_speed Subsystem1/2(yaw_circle_out) -> yaw_circle_out/1
  yaw_status/1 -> Switch Case/1
  yaw_circle/1 -> If Action_speed Subsystem1/5(yaw_circle)
  If Action_speed Subsystem/1(Out1) -> yaw_SPD_OUT/1
  If Action_speed Subsystem1/1(Out1) -> yaw_ANG_OUT/1

== system PID_MODEL/Yaw_CH1_5 ==
  yaw_speed_rpm : Inport  OutDataTypeStr=single
  yaw_target : Inport  Port=2  OutDataTypeStr=single
  yaw_status : Inport  Port=3  OutDataTypeStr=single
  yaw_ecd : Inport  Port=4  OutDataTypeStr=single
  yaw_last_ecd : Inport  Port=5  OutDataTypeStr=single
  yaw_circle : Inport  Port=6  OutDataTypeStr=single
  If Action_speed Subsystem : Subsystem  TreatAsAtomicUnit=on
  If Action_speed Subsystem1 : Subsystem  TreatAsAtomicUnit=on
  Switch Case : SwitchCase  CaseConditions={1,2}  ShowDefaultCase=off
  yaw_SPD_OUT : Outport  OutDataTypeStr=single
  yaw_ANG_OUT : Outport  Port=2  OutDataTypeStr=single
  yaw_circle_out : Outport  Port=3  OutDataTypeStr=single
  wires:
  Switch Case/1 -> If Action_speed Subsystem/Action
  yaw_speed_rpm/1 -> If Action_speed Subsystem1/1(yaw_speed_rpm), If Action_speed Subsystem/1(yaw_speed_rpm)
  yaw_target/1 -> If Action_speed Subsystem1/2(yaw_target), If Action_speed Subsystem/2(yaw_target)
  Switch Case/2 -> If Action_speed Subsystem1/Action
  yaw_ecd/1 -> If Action_speed Subsystem1/3(yaw_ecd)
  yaw_last_ecd/1 -> If Action_speed Subsystem1/4(yaw_last_ecd)
  If Action_speed Subsystem1/2(yaw_circle_out) -> yaw_circle_out/1
  yaw_status/1 -> Switch Case/1
  yaw_circle/1 -> If Action_speed Subsystem1/5(yaw_circle)
  If Action_speed Subsystem/1(Out1) -> yaw_SPD_OUT/1
  If Action_speed Subsystem1/1(Out1) -> yaw_ANG_OUT/1

== system PID_MODEL/Yaw_CH1_6 ==
  yaw_speed_rpm : Inport  OutDataTypeStr=single
  yaw_target : Inport  Port=2  OutDataTypeStr=single
  yaw_status : Inport  Port=3  OutDataTypeStr=single
  yaw_ecd : Inport  Port=4  OutDataTypeStr=single
  yaw_last_ecd : Inport  Port=5  OutDataTypeStr=single
  yaw_circle : Inport  Port=6  OutDataTypeStr=single
  If Action_speed Subsystem : Subsystem  TreatAsAtomicUnit=on
  If Action_speed Subsystem1 : Subsystem  TreatAsAtomicUnit=on
  Switch Case : SwitchCase  CaseConditions={1,2}  ShowDefaultCase=off
  yaw_SPD_OUT : Outport  OutDataTypeStr=single
  yaw_ANG_OUT : Outport  Port=2  OutDataTypeStr=single
  yaw_circle_out : Outport  Port=3  OutDataTypeStr=single
  wires:
  Switch Case/1 -> If Action_speed Subsystem/Action
  yaw_speed_rpm/1 -> If Action_speed Subsystem1/1(yaw_speed_rpm), If Action_speed Subsystem/1(yaw_speed_rpm)
  yaw_target/1 -> If Action_speed Subsystem1/2(yaw_target), If Action_speed Subsystem/2(yaw_target)
  Switch Case/2 -> If Action_speed Subsystem1/Action
  yaw_ecd/1 -> If Action_speed Subsystem1/3(yaw_ecd)
  yaw_last_ecd/1 -> If Action_speed Subsystem1/4(yaw_last_ecd)
  If Action_speed Subsystem1/2(yaw_circle_out) -> yaw_circle_out/1
  yaw_status/1 -> Switch Case/1
  yaw_circle/1 -> If Action_speed Subsystem1/5(yaw_circle)
  If Action_speed Subsystem/1(Out1) -> yaw_SPD_OUT/1
  If Action_speed Subsystem1/1(Out1) -> yaw_ANG_OUT/1

== system PID_MODEL/Yaw_CH1_7 ==
  yaw_speed_rpm : Inport  OutDataTypeStr=single
  yaw_target : Inport  Port=2  OutDataTypeStr=single
  yaw_status : Inport  Port=3  OutDataTypeStr=single
  yaw_ecd : Inport  Port=4  OutDataTypeStr=single
  yaw_last_ecd : Inport  Port=5  OutDataTypeStr=single
  yaw_circle : Inport  Port=6  OutDataTypeStr=single
  If Action_speed Subsystem : Subsystem  TreatAsAtomicUnit=on
  If Action_speed Subsystem1 : Subsystem  TreatAsAtomicUnit=on
  Switch Case : SwitchCase  CaseConditions={1,2}  ShowDefaultCase=off
  yaw_SPD_OUT : Outport  OutDataTypeStr=single
  yaw_ANG_OUT : Outport  Port=2  OutDataTypeStr=single
  yaw_circle_out : Outport  Port=3  OutDataTypeStr=single
  wires:
  Switch Case/1 -> If Action_speed Subsystem/Action
  yaw_speed_rpm/1 -> If Action_speed Subsystem1/1(yaw_speed_rpm), If Action_speed Subsystem/1(yaw_speed_rpm)
  yaw_target/1 -> If Action_speed Subsystem1/2(yaw_target), If Action_speed Subsystem/2(yaw_target)
  Switch Case/2 -> If Action_speed Subsystem1/Action
  yaw_ecd/1 -> If Action_speed Subsystem1/3(yaw_ecd)
  yaw_last_ecd/1 -> If Action_speed Subsystem1/4(yaw_last_ecd)
  If Action_speed Subsystem1/2(yaw_circle_out) -> yaw_circle_out/1
  yaw_status/1 -> Switch Case/1
  yaw_circle/1 -> If Action_speed Subsystem1/5(yaw_circle)
  If Action_speed Subsystem/1(Out1) -> yaw_SPD_OUT/1
  If Action_speed Subsystem1/1(Out1) -> yaw_ANG_OUT/1

== system PID_MODEL/Yaw_CH2_1 ==
  yaw_speed_rpm : Inport  OutDataTypeStr=single
  yaw_target : Inport  Port=2  OutDataTypeStr=single
  yaw_status : Inport  Port=3  OutDataTypeStr=single
  yaw_ecd : Inport  Port=4  OutDataTypeStr=single
  yaw_last_ecd : Inport  Port=5  OutDataTypeStr=single
  yaw_circle : Inport  Port=6  OutDataTypeStr=single
  If Action_speed Subsystem : Subsystem  TreatAsAtomicUnit=on
  If Action_speed Subsystem1 : Subsystem  TreatAsAtomicUnit=on
  Switch Case : SwitchCase  CaseConditions={1,2}  ShowDefaultCase=off
  yaw_SPD_OUT : Outport  OutDataTypeStr=single
  yaw_ANG_OUT : Outport  Port=2  OutDataTypeStr=single
  yaw_circle_out : Outport  Port=3  OutDataTypeStr=single
  wires:
  Switch Case/1 -> If Action_speed Subsystem/Action
  yaw_speed_rpm/1 -> If Action_speed Subsystem1/1(yaw_speed_rpm), If Action_speed Subsystem/1(yaw_speed_rpm)
  yaw_target/1 -> If Action_speed Subsystem1/2(yaw_target), If Action_speed Subsystem/2(yaw_target)
  Switch Case/2 -> If Action_speed Subsystem1/Action
  yaw_ecd/1 -> If Action_speed Subsystem1/3(yaw_ecd)
  yaw_last_ecd/1 -> If Action_speed Subsystem1/4(yaw_last_ecd)
  If Action_speed Subsystem1/2(yaw_circle_out) -> yaw_circle_out/1
  yaw_status/1 -> Switch Case/1
  yaw_circle/1 -> If Action_speed Subsystem1/5(yaw_circle)
  If Action_speed Subsystem/1(Out1) -> yaw_SPD_OUT/1
  If Action_speed Subsystem1/1(Out1) -> yaw_ANG_OUT/1

== system PID_MODEL/Yaw_CH2_2 ==
  yaw_speed_rpm : Inport  OutDataTypeStr=single
  yaw_target : Inport  Port=2  OutDataTypeStr=single
  yaw_status : Inport  Port=3  OutDataTypeStr=single
  yaw_ecd : Inport  Port=4  OutDataTypeStr=single
  yaw_last_ecd : Inport  Port=5  OutDataTypeStr=single
  yaw_circle : Inport  Port=6  OutDataTypeStr=single
  If Action_speed Subsystem : Subsystem  TreatAsAtomicUnit=on
  If Action_speed Subsystem1 : Subsystem  TreatAsAtomicUnit=on
  Switch Case : SwitchCase  CaseConditions={1,2}  ShowDefaultCase=off
  yaw_SPD_OUT : Outport  OutDataTypeStr=single
  yaw_ANG_OUT : Outport  Port=2  OutDataTypeStr=single
  yaw_circle_out : Outport  Port=3  OutDataTypeStr=single
  wires:
  Switch Case/1 -> If Action_speed Subsystem/Action
  yaw_speed_rpm/1 -> If Action_speed Subsystem1/1(yaw_speed_rpm), If Action_speed Subsystem/1(yaw_speed_rpm)
  yaw_target/1 -> If Action_speed Subsystem1/2(yaw_target), If Action_speed Subsystem/2(yaw_target)
  Switch Case/2 -> If Action_speed Subsystem1/Action
  yaw_ecd/1 -> If Action_speed Subsystem1/3(yaw_ecd)
  yaw_last_ecd/1 -> If Action_speed Subsystem1/4(yaw_last_ecd)
  If Action_speed Subsystem1/2(yaw_circle_out) -> yaw_circle_out/1
  yaw_status/1 -> Switch Case/1
  yaw_circle/1 -> If Action_speed Subsystem1/5(yaw_circle)
  If Action_speed Subsystem/1(Out1) -> yaw_SPD_OUT/1
  If Action_speed Subsystem1/1(Out1) -> yaw_ANG_OUT/1

== system PID_MODEL/Yaw_CH2_3 ==
  yaw_speed_rpm : Inport  OutDataTypeStr=single
  yaw_target : Inport  Port=2  OutDataTypeStr=single
  yaw_status : Inport  Port=3  OutDataTypeStr=single
  yaw_ecd : Inport  Port=4  OutDataTypeStr=single
  yaw_last_ecd : Inport  Port=5  OutDataTypeStr=single
  yaw_circle : Inport  Port=6  OutDataTypeStr=single
  If Action_speed Subsystem : Subsystem  TreatAsAtomicUnit=on
  If Action_speed Subsystem1 : Subsystem  TreatAsAtomicUnit=on
  Switch Case : SwitchCase  CaseConditions={1,2}  ShowDefaultCase=off
  yaw_SPD_OUT : Outport  OutDataTypeStr=single
  yaw_ANG_OUT : Outport  Port=2  OutDataTypeStr=single
  yaw_circle_out : Outport  Port=3  OutDataTypeStr=single
  wires:
  Switch Case/1 -> If Action_speed Subsystem/Action
  yaw_speed_rpm/1 -> If Action_speed Subsystem1/1(yaw_speed_rpm), If Action_speed Subsystem/1(yaw_speed_rpm)
  yaw_target/1 -> If Action_speed Subsystem1/2(yaw_target), If Action_speed Subsystem/2(yaw_target)
  Switch Case/2 -> If Action_speed Subsystem1/Action
  yaw_ecd/1 -> If Action_speed Subsystem1/3(yaw_ecd)
  yaw_last_ecd/1 -> If Action_speed Subsystem1/4(yaw_last_ecd)
  If Action_speed Subsystem1/2(yaw_circle_out) -> yaw_circle_out/1
  yaw_status/1 -> Switch Case/1
  yaw_circle/1 -> If Action_speed Subsystem1/5(yaw_circle)
  If Action_speed Subsystem/1(Out1) -> yaw_SPD_OUT/1
  If Action_speed Subsystem1/1(Out1) -> yaw_ANG_OUT/1

== system PID_MODEL/Yaw_CH2_4 ==
  yaw_speed_rpm : Inport  OutDataTypeStr=single
  yaw_target : Inport  Port=2  OutDataTypeStr=single
  yaw_status : Inport  Port=3  OutDataTypeStr=single
  yaw_ecd : Inport  Port=4  OutDataTypeStr=single
  yaw_last_ecd : Inport  Port=5  OutDataTypeStr=single
  yaw_circle : Inport  Port=6  OutDataTypeStr=single
  If Action_speed Subsystem : Subsystem  TreatAsAtomicUnit=on
  If Action_speed Subsystem1 : Subsystem  TreatAsAtomicUnit=on
  Switch Case : SwitchCase  CaseConditions={1,2}  ShowDefaultCase=off
  yaw_SPD_OUT : Outport  OutDataTypeStr=single
  yaw_ANG_OUT : Outport  Port=2  OutDataTypeStr=single
  yaw_circle_out : Outport  Port=3  OutDataTypeStr=single
  wires:
  Switch Case/1 -> If Action_speed Subsystem/Action
  yaw_speed_rpm/1 -> If Action_speed Subsystem1/1(yaw_speed_rpm), If Action_speed Subsystem/1(yaw_speed_rpm)
  yaw_target/1 -> If Action_speed Subsystem1/2(yaw_target), If Action_speed Subsystem/2(yaw_target)
  Switch Case/2 -> If Action_speed Subsystem1/Action
  yaw_ecd/1 -> If Action_speed Subsystem1/3(yaw_ecd)
  yaw_last_ecd/1 -> If Action_speed Subsystem1/4(yaw_last_ecd)
  If Action_speed Subsystem1/2(yaw_circle_out) -> yaw_circle_out/1
  yaw_status/1 -> Switch Case/1
  yaw_circle/1 -> If Action_speed Subsystem1/5(yaw_circle)
  If Action_speed Subsystem/1(Out1) -> yaw_SPD_OUT/1
  If Action_speed Subsystem1/1(Out1) -> yaw_ANG_OUT/1

== system PID_MODEL/Yaw_CH2_5 ==
  yaw_speed_rpm : Inport  OutDataTypeStr=single
  yaw_target : Inport  Port=2  OutDataTypeStr=single
  yaw_status : Inport  Port=3  OutDataTypeStr=single
  yaw_ecd : Inport  Port=4  OutDataTypeStr=single
  yaw_last_ecd : Inport  Port=5  OutDataTypeStr=single
  yaw_circle : Inport  Port=6  OutDataTypeStr=single
  If Action_speed Subsystem : Subsystem  TreatAsAtomicUnit=on
  If Action_speed Subsystem1 : Subsystem  TreatAsAtomicUnit=on
  Switch Case : SwitchCase  CaseConditions={1,2}  ShowDefaultCase=off
  yaw_SPD_OUT : Outport  OutDataTypeStr=single
  yaw_ANG_OUT : Outport  Port=2  OutDataTypeStr=single
  yaw_circle_out : Outport  Port=3  OutDataTypeStr=single
  wires:
  Switch Case/1 -> If Action_speed Subsystem/Action
  yaw_speed_rpm/1 -> If Action_speed Subsystem1/1(yaw_speed_rpm), If Action_speed Subsystem/1(yaw_speed_rpm)
  yaw_target/1 -> If Action_speed Subsystem1/2(yaw_target), If Action_speed Subsystem/2(yaw_target)
  Switch Case/2 -> If Action_speed Subsystem1/Action
  yaw_ecd/1 -> If Action_speed Subsystem1/3(yaw_ecd)
  yaw_last_ecd/1 -> If Action_speed Subsystem1/4(yaw_last_ecd)
  If Action_speed Subsystem1/2(yaw_circle_out) -> yaw_circle_out/1
  yaw_status/1 -> Switch Case/1
  yaw_circle/1 -> If Action_speed Subsystem1/5(yaw_circle)
  If Action_speed Subsystem/1(Out1) -> yaw_SPD_OUT/1
  If Action_speed Subsystem1/1(Out1) -> yaw_ANG_OUT/1

== system PID_MODEL/Yaw_CH2_6 ==
  yaw_speed_rpm : Inport  OutDataTypeStr=single
  yaw_target : Inport  Port=2  OutDataTypeStr=single
  yaw_status : Inport  Port=3  OutDataTypeStr=single
  yaw_ecd : Inport  Port=4  OutDataTypeStr=single
  yaw_last_ecd : Inport  Port=5  OutDataTypeStr=single
  yaw_circle : Inport  Port=6  OutDataTypeStr=single
  If Action_speed Subsystem : Subsystem  TreatAsAtomicUnit=on
  If Action_speed Subsystem1 : Subsystem  TreatAsAtomicUnit=on
  Switch Case : SwitchCase  CaseConditions={1,2}  ShowDefaultCase=off
  yaw_SPD_OUT : Outport  OutDataTypeStr=single
  yaw_ANG_OUT : Outport  Port=2  OutDataTypeStr=single
  yaw_circle_out : Outport  Port=3  OutDataTypeStr=single
  wires:
  Switch Case/1 -> If Action_speed Subsystem/Action
  yaw_speed_rpm/1 -> If Action_speed Subsystem1/1(yaw_speed_rpm), If Action_speed Subsystem/1(yaw_speed_rpm)
  yaw_target/1 -> If Action_speed Subsystem1/2(yaw_target), If Action_speed Subsystem/2(yaw_target)
  Switch Case/2 -> If Action_speed Subsystem1/Action
  yaw_ecd/1 -> If Action_speed Subsystem1/3(yaw_ecd)
  yaw_last_ecd/1 -> If Action_speed Subsystem1/4(yaw_last_ecd)
  If Action_speed Subsystem1/2(yaw_circle_out) -> yaw_circle_out/1
  yaw_status/1 -> Switch Case/1
  yaw_circle/1 -> If Action_speed Subsystem1/5(yaw_circle)
  If Action_speed Subsystem/1(Out1) -> yaw_SPD_OUT/1
  If Action_speed Subsystem1/1(Out1) -> yaw_ANG_OUT/1

== system PID_MODEL/Yaw_CH2_7 ==
  yaw_speed_rpm : Inport  OutDataTypeStr=single
  yaw_target : Inport  Port=2  OutDataTypeStr=single
  yaw_status : Inport  Port=3  OutDataTypeStr=single
  yaw_ecd : Inport  Port=4  OutDataTypeStr=single
  yaw_last_ecd : Inport  Port=5  OutDataTypeStr=single
  yaw_circle : Inport  Port=6  OutDataTypeStr=single
  If Action_speed Subsystem : Subsystem  TreatAsAtomicUnit=on
  If Action_speed Subsystem1 : Subsystem  TreatAsAtomicUnit=on
  Switch Case : SwitchCase  CaseConditions={1,2}  ShowDefaultCase=off
  yaw_SPD_OUT : Outport  OutDataTypeStr=single
  yaw_ANG_OUT : Outport  Port=2  OutDataTypeStr=single
  yaw_circle_out : Outport  Port=3  OutDataTypeStr=single
  wires:
  Switch Case/1 -> If Action_speed Subsystem/Action
  yaw_speed_rpm/1 -> If Action_speed Subsystem1/1(yaw_speed_rpm), If Action_speed Subsystem/1(yaw_speed_rpm)
  yaw_target/1 -> If Action_speed Subsystem1/2(yaw_target), If Action_speed Subsystem/2(yaw_target)
  Switch Case/2 -> If Action_speed Subsystem1/Action
  yaw_ecd/1 -> If Action_speed Subsystem1/3(yaw_ecd)
  yaw_last_ecd/1 -> If Action_speed Subsystem1/4(yaw_last_ecd)
  If Action_speed Subsystem1/2(yaw_circle_out) -> yaw_circle_out/1
  yaw_status/1 -> Switch Case/1
  yaw_circle/1 -> If Action_speed Subsystem1/5(yaw_circle)
  If Action_speed Subsystem/1(Out1) -> yaw_SPD_OUT/1
  If Action_speed Subsystem1/1(Out1) -> yaw_ANG_OUT/1

== system PID_MODEL/Yaw_CH1_1/If Action_speed Subsystem ==
  yaw_speed_rpm : Inport  OutDataTypeStr=single
  yaw_target : Inport  Port=2  OutDataTypeStr=single
  Action Port : ActionPort  ActionPortLabel=case [ 1 ]:
  Discrete PID Controller1 : slpidlib/PID Controller  Controller=PID  Form=Parallel  TimeDomain=Discrete-time  UseExternalTs=off  SampleTime=-1  IntegratorMethod=Forward Euler  FilterMethod=Forward Euler  ControllerParametersSource=internal  P=SPD_P_CH1_1  I=SPD_I_CH1_1  UseKiTs=off  D=SPD_D_CH1_1  N=100  UseFilter=on  TunerSelectOption=Transfer Function Based (PID Tuner App)  InitialConditionSource=internal  InitialConditionForIntegrator=0  InitialConditionForFilter=0  DifferentiatorICPrevScaledInput=0  ExternalReset=none  TrackingMode=off  Kt=1  LimitOutput=on  SatLimitsSource=internal  UpperSaturationLimit=16384  LowerSaturationLimit=-16384  LinearizeAsGain=off  AntiWindupMode=none  Kb=1  LimitIntegrator=off  UpperIntegratorSaturationLimit=inf  LowerIntegratorSaturationLimit=-inf  POutMin=[]  POutMax=[]  IOutMin=[]  IOutMax=[]  DOutMin=[]  DOutMax=[]  NOutMin=[]  NOutMax=[]  SumOutMin=[]  SumOutMax=[]  SaturationOutMin=[]  SaturationOutMax=[]  PParamMin=[]  PParamMax=[]  IParamMin=[]  IParamMax=[]  DParamMin=[]  DParamMax=[]  NParamMin=[]  NParamMax=[]  KbParamMin=[]  KbParamMax=[]  KtParamMin=[]  KtParamMax=[]  KbOutMin=[]  KbOutMax=[]  KtOutMin=[]  KtOutMax=[]  IntegratorOutMin=[]  IntegratorOutMax=[]  FilterOutMin=[]  FilterOutMax=[]  SumI1OutMin=[]  SumI1OutMax=[]  SumI2OutMin=[]  SumI2OutMax=[]  SumI3OutMin=[]  SumI3OutMax=[]  SumI4OutMin=[]  SumI4OutMax=[]  SumDOutMin=[]  SumDOutMax=[]  DifferentiatorOutMin=[]  DifferentiatorOutMax=[]  FilterDiffOutCoefMin=[]  FilterDiffOutCoefMax=[]  ReciprocalOutMin=[]  ReciprocalOutMax=[]  SumDenOutMin=[]  SumDenOutMax=[]  SumNumOutMin=[]  SumNumOutMax=[]  DivideOutMin=[]  DivideOutMax=[]  UdiffTsProdOutMin=[]  UdiffTsProdOutMax=[]  NTsProdOutMin=[]  NTsProdOutMax=[]  UintegralTsProdOutMin=[]  UintegralTsProdOutMax=[]  UngainTsProdOutMin=[]  UngainTsProdOutMax=[]  ClampingZeroOutDataTypeStr=Inherit: Inherit via back propagation  ClampingZeroOutMin=[]  ClampingZeroOutMax=[]  FilterDenConstantOutDataTypeStr=Inherit: Inherit via back propagation  FilterDenConstantOutMin=[]  FilterDenConstantOutMax=[]  PCopyOutDataTypeStr=Inherit: Inherit via back propagation  PCopyOutMin=[]  PCopyOutMax=[]  NCopyOutDataTypeStr=Inherit: Inherit via back propagation  NCopyOutMin=[]  NCopyOutMax=[]  IntegratorContinuousStateAttributes=''  IntegratorStateMustResolveToSignalObject=off  IntegratorRTWStateStorageClass=Auto  FilterContinuousStateAttributes=''  FilterStateMustResolveToSignalObject=off  FilterRTWStateStorageClass=Auto  ParallelPVariant=InternalParameters  IdealPVariant=Disabled  IVariant=InternalParameters  DVariant=InternalParameters  IntegratorVariant=Discrete  SatVariant=Enabled  AWVariant=Passthrough  PCopyVariant=Disabled  TRVariant=Disabled  FdbkBlocksVariant=Forward  IdealPFdbkVariant=Disabled  SatFdbkVariant=Disabled  DerivativeFilterVariant=ForwardEulerFilter  NVariant=InternalParameters  NCopyVariant=Disabled  FilterICVariant=InternalICsFilter  IntegratorICVariant=InternalICs  ExternalResetVariant=Disabled  TRSumVariant=Passthrough  SumFdbkVariant=Disabled  SumVariant=Sum_PID  TsampFilterVariant=InternalTs  TsampNgainVariant=Passthrough  TsampIntegralVariant=Disabled_SignalSpec  ExternalSaturationOutDataTypeStr=Inherit: Same as second input
      settings: LibrarySourceBlock=simulink/Discrete/Discrete PID Controller
  Sum : Sum  Inputs=|+-  OutDataTypeStr=single
  Out1 : Outport  OutDataTypeStr=single
  wires:
  yaw_speed_rpm/1 -> Sum/2
  yaw_target/1 -> Sum/1
  Sum/1 -> Discrete PID Controller1/1
  Discrete PID Controller1/1 -> Out1/1
